simulink model "forward_kinematics_model"  (R2025a)
settings: Solver=FixedStepAuto  StartTime=0.0  StopTime=40  FixedStep=0.001  RelTol=1e-3  EnableMultiTasking=on
settings Model: SILPILModeSetting=veronly  ExtModeTrigDuration=2  Creator=jonas  LastModifiedBy=zafi
settings SolverCC: AllowMultiTaskInputOutput=on  ConcurrentTasks=on
settings OptimizationCC: DefaultUnderspecifiedDataType=single  EnhancedBackFolding=on  PassReuseOutputArgsAs=Individual arguments  ZeroExternalMemoryAtStartup=off  ZeroInternalMemoryAtStartup=off  EfficientFloat2IntCast=on  MaxStackSize=64  SimCompilerOptimization=on  OptimizeBlockOrder=speed  DifferentSizesBufferReuse=on  OptimizationCustomize=off  EfficientTunableParamExpr=on
settings DebuggingCC: ParameterTunabilityLossMsg=error
settings HardwareCC: ProdBitPerInt=16.0  ProdBitPerPointer=16.0  ProdBitPerSizeT=16.0  ProdBitPerPtrDiffT=16.0  ProdLargestAtomicFloat=None  ProdWordSize=8.0  ProdHWDeviceType=Atmel->AVR
settings ModelReferenceCC: EnableParallelModelReferenceBuilds=on  ModelReferenceMinAlgLoopOccurrences=on
settings SFSimCC: MATLABDynamicMemAllocThreshold=32000.0  SimTargetLang=C++  SimDLTargetLibrary=mkl-dnn
settings RTWCC: SystemTargetFile=ert.tlc  HardwareBoard=Arduino Mega 2560  TemplateMakefile=ert_default_tmf  Toolchain=Arduino AVR  BuildConfiguration=Faster Runs  GPUComputeCapability=3.5  Description=Embedded Coder
settings CodeAppCC: ForceParamTrailComments=on  IgnoreCustomStorageClasses=off  OperatorAnnotations=on  SimulinkDataObjDesc=on  SFDataObjDesc=on  InsertBlockDesc=on
settings ERTTargetCC: ExtModeTransport=3.0  ExtModeAutomaticAllocSize=off  ExtModeStaticAllocSize=2048.0  InlinedParameterPlacement=Hierarchical  DynamicArrayContainerType=coder::array  SupportContinuousTime=on  SupportVariableSizeSignals=on

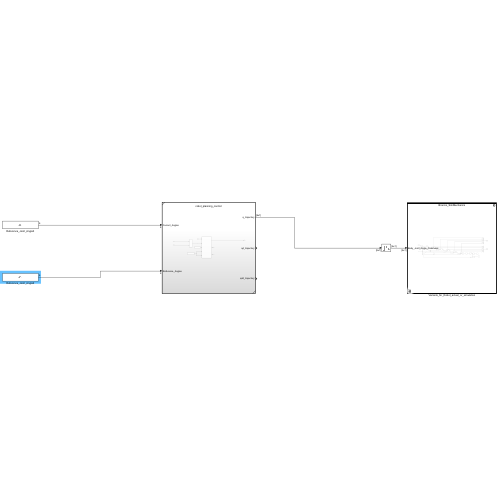
[thumbnail: Simulink's stored preview of the top-level diagram]
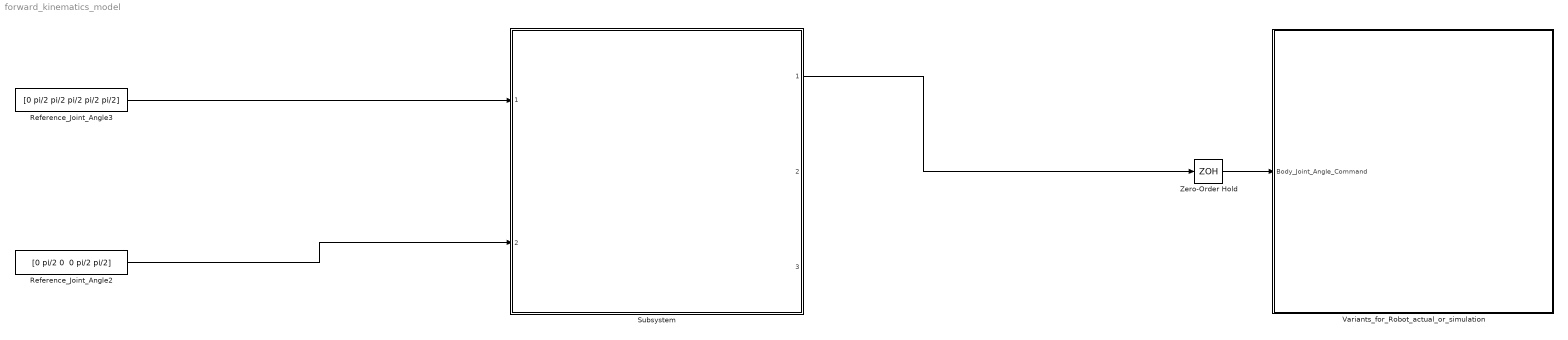
== system forward_kinematics_model ==
  Reference_Joint_Angle2 : Constant  Value="[0 pi/2 0  0 pi/2 pi/2]"
  Reference_Joint_Angle3 : Constant  Value=[0 pi/2 pi/2 pi/2 pi/2 pi/2]
  Subsystem : Subsystem  TreatAsAtomicUnit=on  ReferencedSubsystem=robot_planning_control
  Variants_for_Robot_actual_or_simulation : Subsystem  TreatAsAtomicUnit=on  Variant=on  VariantChoicesSpecifier={'Braccio_Arduino', 'Braccio_SimMechanics'}  VariantControlMode=label  VariantControl=Choice  LabelModeActiveChoice=Braccio_SimMechanics
  Zero-Order Hold : ZeroOrderHold  SampleTime=-1
  wires:
  Zero-Order Hold/1 -> Variants_for_Robot_actual_or_simulation/1(Body_Joint_Angle_Command)
  Subsystem/1 -> Zero-Order Hold/1
  Reference_Joint_Angle3/1 -> Subsystem/1
  Reference_Joint_Angle2/1 -> Subsystem/2

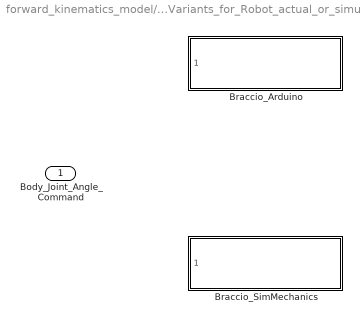
== system forward_kinematics_model/Variants_for_Robot_actual_or_simulation ==
  Body_Joint_Angle_Command : Inport
  Braccio_Arduino : Subsystem  TreatAsAtomicUnit=on  VariantControl=Braccio_Arduino  ReferencedSubsystem=Braccio_Arduino
  Braccio_SimMechanics : Subsystem  TreatAsAtomicUnit=on  VariantControl=Braccio_SimMechanics  ReferencedSubsystem=Braccio_SimMechanics
